simulink model "test_poisson"  (Simulink 7.7)
settings: Solver=ode45  StartTime=0.0  StopTime=10.0  RelTol=1e-3
undefined symbols (not defined in the file): des_attributefunction_support, des_figposition
libraries: simeventssink1 x5, simeventsattributes2 x3, commrandsrc2 x3, simeventsgenerators1 x2, simeventstranslate1 x1, simeventsqueue1 x1, simeventsserver1 x1
settings Model: Creator=german  LastModifiedBy=german
settings SimEventsCC: propDiagAttribOutput=1  propDiagFcnCallOutput=1  propDiagStatOutput=0

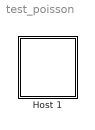
== system test_poisson ==
  Host 1 : Subsystem

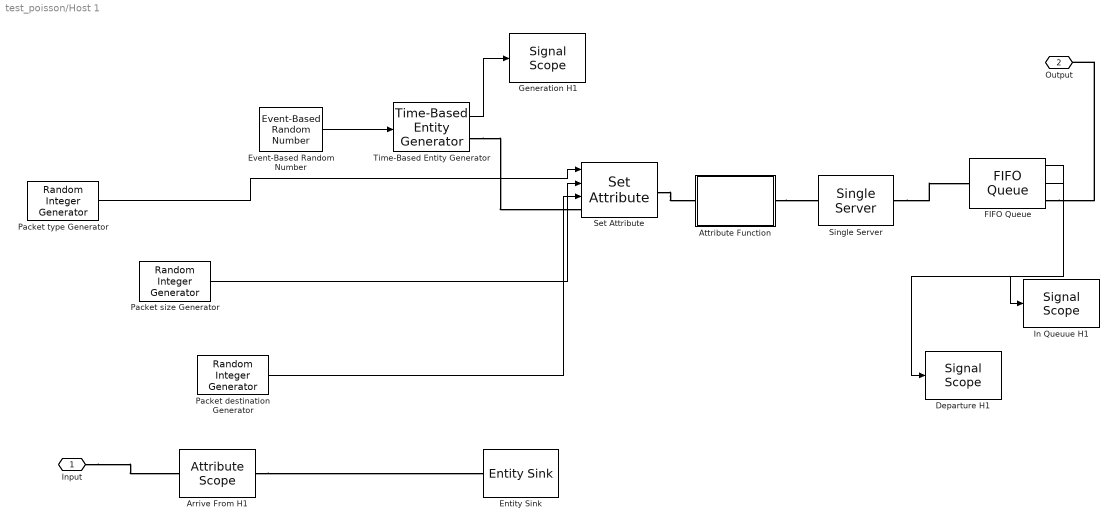
== system test_poisson/Host 1 ==
  Arrive From H1 : simeventssink1/Attribute Scope  SystemSampleTime=-1  PlotType=Stair  InputType=Attribute  NumInputs=1  AttributeNameY=from  XInputOptionSignal=Event time  XInputOptionEntity=Event time  AttributeNameX=Count  EnableEntityOutport=on  XMin=0  XMax=10  XLimitExceededOption=Stretch axis limits  YLimitExceededOption=Stretch axis limits  AxisGrid=on  AxisLegend=off  LineDisables=""  LineColors=b  LineStyles=-  LineMarkers=.  OpenScopeAtSimStart=on  Title=""  YLabel=""  XLabel=Time  FigurePosition=des_figposition([5 25 25 25])  AxisZoom=off  DataStoreOption=Limited  DataPointsLimit=10000  StatNumberArrived=Off  ShowCountPlotted=off  ShowToolbar=on
      settings: YMin=0  YMax=10
  Attribute Function : Subsystem  LoadFcn=des_attributefunction_support(gcb,'LoadFcn');  StartFcn=des_attributefunction_support(gcb,'StartFcn');  mask(Attribute Function){OutputNamePrefix=out_}
      mask prompts: OutputNamePrefix "Prefix name"
      settings: CopyFcn=des_attributefunction_support(gcb,'CopyFcn');  OpenFcn=des_attributefunction_support(gcb,'OpenFcn');  ErrorFcn=des_error_redirect
      mask Help: helpview(simeventsbhelp('attributefunction'))
      mask Display: image(des_iconLoad('attribFunction.jpg'),'center');
  Departure H1 : simeventssink1/Signal Scope  SystemSampleTime=-1  PlotType=Stair  InputType=Signal  NumInputs=1  AttributeNameY=Count  XInputOptionSignal=Event time  XInputOptionEntity=Event time  AttributeNameX=Count  EnableEntityOutport=on  XMin=0  XMax=10  XLimitExceededOption=Stretch axis limits  YLimitExceededOption=Stretch axis limits  AxisGrid=on  AxisLegend=off  LineDisables=""  LineColors=b  LineStyles=-  LineMarkers=.  OpenScopeAtSimStart=on  Title=""  YLabel=""  XLabel=Time  FigurePosition=des_figposition([5 60 25 25])  AxisZoom=off  DataStoreOption=Limited  DataPointsLimit=10000  StatNumberArrived=Off  ShowCountPlotted=off  ShowToolbar=on
      settings: YMin=0  YMax=10
  Entity Sink : simeventssink1/Entity Sink  SystemSampleTime=-1  AvailableForArrivals=on  StatNumberArrived=On
  Event-Based Random Number : simeventsgenerators1/Signal Generators/Event-Based Random Number  SystemSampleTime=-1  distribution=Poisson  meanExp=1  minUnif=1  maxUnif=1  pOneBern=0.25  pSuccessBino=0.5  numTrialBino=1  meanNorm=0  stdNorm=1  minTri=1  maxTri=3  modeTri=2  thresholdLogn=0  scaleLogn=1  shapeLogn=1  pSuccessGeo=0.5  meanPoiss=0.1  thresholdLogl=0  scaleLogl=1  thresholdGam=0  scaleGam=1  shapeGam=1  minBeta=0  maxBeta=1  shape1Beta=1  shape2Beta=1  minUnid=0  maxUnid=1  numValueUnid=2  thresholdWbl=0  scaleWbl=1  shapeWbl=1  valueVecCont=[0 1]  cdfVecCont=[0 1]  valueVecDisc=[0 1]  probVecDisc=[0.5 0.5]  seed=12345  IsProcessed=on  isConnected=1
  FIFO Queue : simeventsqueue1/FIFO Queue  SystemSampleTime=-1  Capacity=25  EnableTOPort=off  StatNumberDeparted=On  StatNumberInBlock=On  StatPendingEntity=Off  StatAverageWait=Off  StatAverageQueueLength=Off  StatNumberTimedout=Off
  Generation H1 : simeventssink1/Signal Scope  SystemSampleTime=-1  PlotType=Stair  InputType=Signal  NumInputs=1  AttributeNameY=Count  XInputOptionSignal=Event time  XInputOptionEntity=Event time  AttributeNameX=Count  EnableEntityOutport=on  XMin=0  XMax=10  XLimitExceededOption=Stretch axis limits  YLimitExceededOption=Stretch axis limits  AxisGrid=on  AxisLegend=off  LineDisables=""  LineColors=b  LineStyles=-  LineMarkers=.  OpenScopeAtSimStart=on  Title=""  YLabel=""  XLabel=Time  FigurePosition=des_figposition([5 60 25 25])  AxisZoom=off  DataStoreOption=Limited  DataPointsLimit=10000  StatNumberArrived=Off  ShowCountPlotted=off  ShowToolbar=on
      settings: YMin=0  YMax=10
  In Queuue H1 : simeventssink1/Signal Scope  SystemSampleTime=-1  PlotType=Stair  InputType=Signal  NumInputs=1  AttributeNameY=Count  XInputOptionSignal=Event time  XInputOptionEntity=Event time  AttributeNameX=Count  EnableEntityOutport=on  XMin=0  XMax=10  XLimitExceededOption=Stretch axis limits  YLimitExceededOption=Stretch axis limits  AxisGrid=on  AxisLegend=off  LineDisables=""  LineColors=b  LineStyles=-  LineMarkers=.  OpenScopeAtSimStart=on  Title=""  YLabel=""  XLabel=Time  FigurePosition=des_figposition([5 60 25 25])  AxisZoom=off  DataStoreOption=Limited  DataPointsLimit=10000  StatNumberArrived=Off  ShowCountPlotted=off  ShowToolbar=on
      settings: YMin=0  YMax=10
  Packet destination Generator : commrandsrc2/Random Integer Generator  SystemSampleTime=-1  mul=6  seed=22  Ts=1  frameBased=off  sampPerFrame=1  orient=off  outDataType=double
  Packet size Generator : commrandsrc2/Random Integer Generator  SystemSampleTime=-1  mul=2  seed=22  Ts=1  frameBased=off  sampPerFrame=1  orient=off  outDataType=double
  Packet type Generator : commrandsrc2/Random Integer Generator  SystemSampleTime=-1  mul=2  seed=37  Ts=1  frameBased=off  sampPerFrame=1  orient=off  outDataType=double
  Set Attribute : simeventsattributes2/Set Attribute  SystemSampleTime=-1  AttributeFrom=Signal port|Signal port|Signal port|Dialog  AttributeName=type|size|dest|from  AttributeTreatAsVector=1|1|1|1  AttributeValue=1|1|4|1  AttributeCreate=on  StatNumberDeparted=Off  EvaluatedAttributeValue={[];[];[];1}
  Single Server : simeventsserver1/Single Server  SystemSampleTime=-1  ServiceTimeFrom=Dialog  ServiceTime=0  AttributeName=ServiceTime  PriorityServiceCompletion=500  PermitPreemption=off  SortingAttributeName=PriorityAttributeName  SortingDirection=Ascending  WriteToAttribute=off  ResidualAttributeName=ResidualServiceTime  CreateAttribute=on  EnableTOPort=off  StatNumberDeparted=Off  StatNumberInBlock=Off  StatNumberPreempted=Off  StatPendingEntity=Off  StatAverageWait=Off  StatUtilization=Off  StatNumberTimedout=Off
  Time-Based Entity Generator : simeventsgenerators1/Entity Generators/Time-Based Entity Generator  SystemSampleTime=-1  GenerateEntitiesUpon=Intergeneration time from port t  Distribution=Constant  Minimum=0  Maximum=1  Mean=1  InitialSeed=12345  Period=1  PriorityEntityGeneration=300  GenerateEntityAtSimulationStart=on  ResponseWhenBlocked=Pause generation  ResponseWhenUnblocked=Immediate restart  EntityType=Standard  StatNumberDeparted=On  StatPendingEntity=Off  StatAverageIntergenerationTime=Off
  Input : PMIOPort  Port=1  Side=Right
  Output : PMIOPort  Port=2  Side=Right
  wires:
  Event-Based Random Number/1 -> Time-Based Entity Generator/1
  Packet size Generator/1 -> Set Attribute/2
  Packet destination Generator/1 -> Set Attribute/3
  FIFO Queue/2 -> In Queuue H1/1
  Packet type Generator/1 -> Set Attribute/1
  FIFO Queue/1 -> Departure H1/1
  Time-Based Entity Generator/1 -> Generation H1/1
  connections:
  Time-Based Entity Generator/RConn1 -- Set Attribute/LConn1
  Set Attribute/RConn1 -- Attribute Function/LConn1
  FIFO Queue/RConn1 -- Output/RConn1
  Attribute Function/RConn1 -- Single Server/LConn1
  Single Server/RConn1 -- FIFO Queue/LConn1
  Input/RConn1 -- Arrive From H1/LConn1
  Arrive From H1/RConn1 -- Entity Sink/LConn1

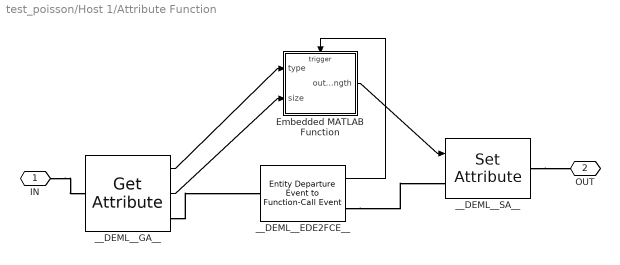
== system test_poisson/Host 1/Attribute Function ==
  Embedded MATLAB Function : Stateflow chart  TreatAsAtomicUnit=on
      settings: PropExecContextOutsideSubsystem=on
  __DEML__EDE2FCE__ : simeventstranslate1/Entity Departure Event to Function-Call Event  Priority=1  SystemSampleTime=-1  TimingFunctionCallF1=Before entity departure  EnableE1Port=off  EnableF2Port=off  TimingFunctionCallF2=Before entity departure  EnableE2Port=off  StatNumberDeparted=Off  StatNumberF1Calls=Off  StatNumberF2Calls=Off  IsInsideAFB=on
  __DEML__GA__ : simeventsattributes2/Get Attribute  Priority=1  SystemSampleTime=-1  AttributeName=type|size  AttributeMissing=Error|Error  AttributeDefaultValue=1|1  AttributeSendTiming=Before entity departure|Before entity departure  AttributeTreatAsVector=1|1  StatNumberDeparted=Off  EvaluatedDefaultAttributeValue={[];[]}
  __DEML__SA__ : simeventsattributes2/Set Attribute  Priority=1  SystemSampleTime=-1  AttributeFrom=Signal port  AttributeName=length  AttributeTreatAsVector=1  AttributeValue=1  AttributeCreate=on  StatNumberDeparted=Off  EvaluatedAttributeValue={[]}
  IN : PMIOPort  Port=1  Side=Left
  OUT : PMIOPort  Port=2  Side=Right
  wires:
  __DEML__EDE2FCE__/1 -> Embedded MATLAB Function/Trigger
  __DEML__GA__/1 -> Embedded MATLAB Function/1(type)
  __DEML__GA__/2 -> Embedded MATLAB Function/2(size)
  Embedded MATLAB Function/1(out_length) -> __DEML__SA__/1
  connections:
  __DEML__SA__/RConn1 -- OUT/RConn1
  IN/RConn1 -- __DEML__GA__/LConn1
  __DEML__GA__/RConn1 -- __DEML__EDE2FCE__/LConn1
  __DEML__EDE2FCE__/RConn1 -- __DEML__SA__/LConn1

== matlab function Host 1/Attribute Function/Embedded MATLAB Function ==
  data: type input double; out_length output double; size input double
  events: trigger input FUNCTION_CALL_EVENT
function out_length  = fcn(type, size)
base = 256;
if (type == 1)
    base = 512;
end
out_length = base * 2^size*8;
